simulink subsystem "Elevation_Deployment"  (R2023b)
settings: Solver=VariableStepAuto  StartTime=0.0  StopTime=10.0  RelTol=1e-3
undefined symbols (not defined in the file): launch_elevation
settings Model: Creator=thatf  LastModifiedBy=thatf

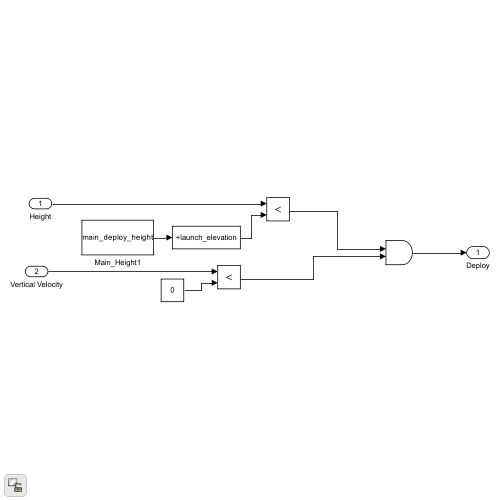
[thumbnail: Simulink's stored preview of the top-level diagram]
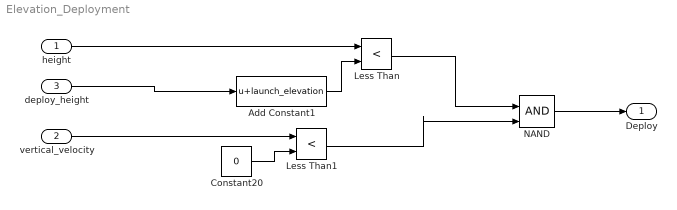
== system Elevation_Deployment ==
  height : Inport
  vertical_velocity : Inport  Port=2
  deploy_height : Inport  Port=3
  Add Constant1 : Bias  Bias=launch_elevation  SaturateOnIntegerOverflow=off
  Constant20 : Constant  Value=0
  Less Than : RelationalOperator  Operator=<  OutDataTypeStr=boolean  RndMeth=Simplest  InputSameDT=off
  Less Than1 : RelationalOperator  Operator=<  OutDataTypeStr=boolean  RndMeth=Simplest  InputSameDT=off
  NAND : Logic  IconShape=distinctive  AllPortsSameDT=off  OutDataTypeStr=boolean
  Deploy : Outport
  wires:
  deploy_height/1 -> Add Constant1/1
  height/1 -> Less Than/1
  Add Constant1/1 -> Less Than/2
  NAND/1 -> Deploy/1
  Less Than1/1 -> NAND/2
  Less Than/1 -> NAND/1
  vertical_velocity/1 -> Less Than1/1
  Constant20/1 -> Less Than1/2
